simulink model "Chap5"  (R2022a)
settings: Solver=VariableStepAuto  StartTime=0.0  StopTime=20  RelTol=1e-3
libraries: Solver_SF x1
settings Model: Creator=陈莹  LastModifiedBy=YiRuQ
settings SolverCC: AlgebraicLoopSolver=TrustRegion
settings DataIOCC: ReturnWorkspaceOutputs=off
settings DebuggingCC: UnconnectedInputMsg=warning  UnconnectedOutputMsg=warning  UnconnectedLineMsg=warning  SFMachineParentedDataDiag=warning  ArithmeticOperatorsInVariantConditions=warning
settings SFSimCC: CustomCodeUndefinedFunction=UseInterfaceOnly
settings RTWCC: DLArmComputeVersion=19.05

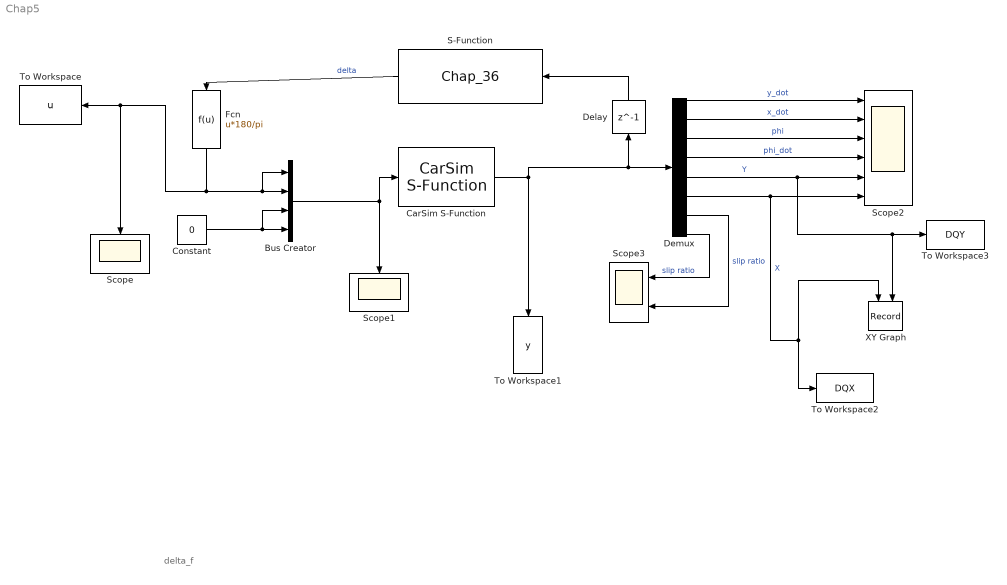
== system Chap5 ==
  note: delta_f
  Bus Creator : BusCreator  Inputs=4
  CarSim S-Function : Solver_SF/CarSim S-Function  Priority=1  SIMFILE=simfile.sim
  Constant : Constant  Value=0
  Delay : Delay  DelayLength=1  InitialCondition=0
  Demux : Demux  Outputs=8
  Fcn : Fcn  Expr=u*180/pi
  S-Function : S-Function  FunctionName=Chap_36  SFunctionDeploymentMode=off  EnableBusSupport=off
  Scope : Scope
  Scope1 : Scope
  Scope2 : Scope  NumInputPorts=6
  Scope3 : Scope  NumInputPorts=2
  To Workspace : ToWorkspace  VariableName=u  SaveFormat=Timeseries  SampleTime=-1
  To Workspace1 : ToWorkspace  VariableName=y  SampleTime=-1
      settings: Save2DSignal=2-D array (concatenate along first dimension)
  To Workspace2 : ToWorkspace  VariableName=DQX  SampleTime=-1
  To Workspace3 : ToWorkspace  VariableName=DQY  SampleTime=-1
  XY Graph : Record  FileSettingsInternal="{\"entries\":[{\"content\":{\"excelSettings\":{\"content\":{},\"type\":\"Streamout.ExcelSettings\"}},\"type\":\"Streamout.FileSettingStorage\",\"uuid\":\"91e1db73-3700-442d-a5f4-9b99973fe8e5\"}],\"packageUris\":[\"http://schema.mathworks.com/mf0/streamout_blocks/R2020a\"],\"version\":\"1.0\"}"  Layout=[1 1]  SignalsInternal="{\"entries\":[{\"content\":{\"signals\":[{\"content\":{\"blockPath\":[\"Chap5/XY Graph\"],\"channel\":[],\"dimensions\":[1],\"domain\":\"Chap5/XY Graph\",\"lineColor\":\"#a2142f\",\"plots\":[1],\"port\":1,\"sid\":[\"\"],\"signalID\":20,\"signalName\":\"X\"},\"type\":\"RecordBlkView.Signal\",\"uuid\":\"575509ca-776c-407e-a085-103da4295aa9\"},{\"content\":{\"blockPath\":[\"Chap5/XY Graph\"],\"channel\":[],\"dimensions\":[1],\"domain\":\"Chap5/XY Graph\",\"lineColor\":\"#139fff\",\"plots\":[1],\"port\":2,\"sid\":[\"\"],\"signalID\":24,\"signalName\":\"Y\"},\"type\":\"RecordBlkView.Signal\",\"uuid\":\"1f22f4cc-1250-4672-bcbd-964b24b9f6f7\"}]},\"type\":\"RecordBlkView.InputSignals\",\"uuid\":\"276d5f03-9b41-4125-ac30-0cf01103e18a\"}],\"packageUris\":[\"http://schema.mathworks.com/mf0/streamout_blocks/R2020a\"],\"version\":\"1.0\"}"  VisualizationBindings="{\"xyplotplugin\":{\"info\":[{\"series\":[{\"bindingParametersList\":[{\"parameter\":\"X-Axis\",\"signalID\":20,\"signalName\":\"X\"},{\"parameter\":\"Y-Axis\",\"signalID\":24,\"signalName\":\"Y\"}],\"seriesID\":17605}],\"subplotID\":1}]}}"  CompatibilityTag=XY  st=-1
  wires:
  Bus Creator/1 -> Scope1/1, CarSim S-Function/1
  Constant/1 -> Bus Creator/4, Bus Creator/3
  Fcn/1 -> Bus Creator/2, Bus Creator/1, Scope/1, To Workspace/1
  S-Function/1 -> Fcn/1  "delta"
  CarSim S-Function/1 -> Delay/1, Demux/1, To Workspace1/1
  Delay/1 -> S-Function/1
  Demux/1 -> Scope2/1  "y_dot"
  Demux/2 -> Scope2/2  "x_dot"
  Demux/3 -> Scope2/3  "phi"
  Demux/4 -> Scope2/4  "phi_dot"
  Demux/5 -> To Workspace3/1, XY Graph/2, Scope2/5  "Y"
  Demux/6 -> Scope2/6, To Workspace2/1, XY Graph/1  "X"
  Demux/7 -> Scope3/2  "slip ratio"
  Demux/8 -> Scope3/1  "slip ratio"
